simulink model "GHV_open_VarialbeMass_toolbox"  (R2023b)
settings: Solver=VariableStepAuto  StartTime=0.0  StopTime=10  FixedStep=0.0000001  MaxStep=0.001  RelTol=1e-3
InitFcn:
  | run('init.m')
values from neighbouring files (symbols this model uses):
  engine_enable = 1    [GHV_Configuration.m]
  GHV_cfg = struct()    [GHV_Configuration.m]
libraries: simulink_extras x3, aerolibtransform2 x3, aerolibasang x3, shared6dof x1, aerolibatmos2 x1
settings Model: SimulationMode=accelerator  Creator=Admin  LastModifiedBy=Admin
settings SolverCC: AllowMultiTaskInputOutput=on  ZeroCrossControl=EnableAll  ZeroCrossAlgorithm=Adaptive  AutoInsertRateTranBlk=on

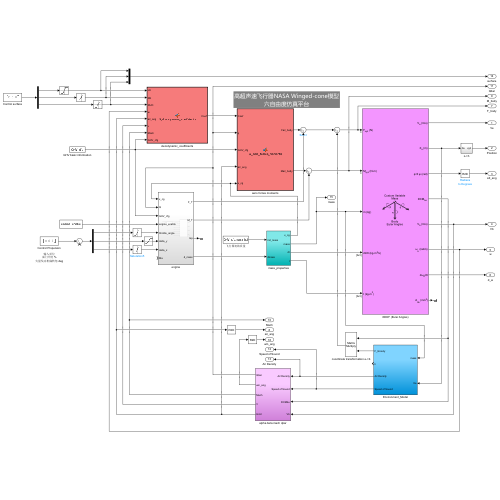
[thumbnail: Simulink's stored preview of the top-level diagram]
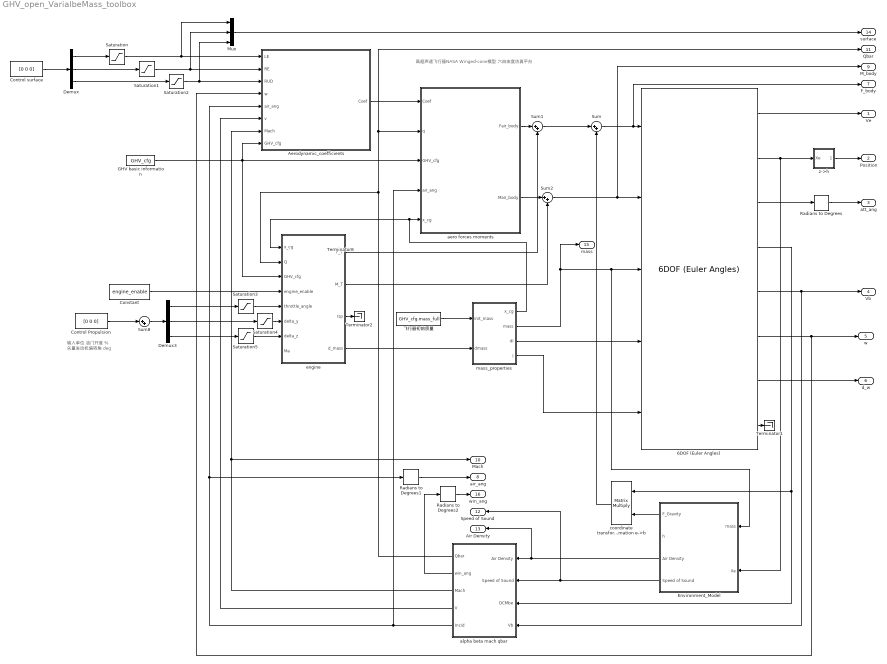
== system GHV_open_VarialbeMass_toolbox ==
  note: 高超声速飞行器NASA Winged-cone模型
      | 六自由度仿真平台
  note: 输入单位
      | 油门开度 %
      | 矢量发动机偏转角 deg
  6DOF (Euler Angles) : shared6dof/6DOF (Euler Angles)  units=Metric (MKS)  mtype=Custom Variable  rep=Euler Angles  xme_0=Position_init  Vm_0=Speed_init  eul_0=Euler_init  pm_0=Omega_init  mass_0=GHV_cfg.mass_full  mass_e=0.5  mass_f=2.0  inertia=GHV_cfg.J  inertia_e=eye(3)  inertia_f=2*eye(3)  k_quat=1.0  vre_flag=off  abi_flag=off  aMode=0  xme_statename=''  Vm_statename=''  eul_statename=''  quat_statename=''  pm_statename=''  mass_statename=''
  Aerodynamic_coefficients : MATLAB Function  TreatAsAtomicUnit=on
  Constant : Constant  Value=engine_enable
  Control Propulsion : Constant  Value=[0 0 0]
  Control surface : Constant  Value=[0 0 0]
  Demux : Demux  Outputs=3
  Demux3 : Demux  Outputs=3
  Environment_Model : Subsystem
  GHV basic information : Constant  Value=GHV_cfg  VectorParams1D=off  OutDataTypeStr=Bus: slBus1
  Mux : Mux  Inputs=3
  Radians to Degrees : simulink_extras/Transformations/Radians to Degrees
  Radians to Degrees1 : simulink_extras/Transformations/Radians to Degrees
  Radians to Degrees2 : simulink_extras/Transformations/Radians to Degrees
  Saturation : Saturate  UpperLimit=30  LowerLimit=-30
  Saturation1 : Saturate  UpperLimit=30  LowerLimit=-30
  Saturation2 : Saturate  UpperLimit=30  LowerLimit=-30
  Saturation3 : Saturate  UpperLimit=52.5  LowerLimit=0  ZeroCross=off
  Saturation4 : Saturate  UpperLimit=10  LowerLimit=-10  ZeroCross=off
  Saturation5 : Saturate  UpperLimit=10  LowerLimit=-10  ZeroCross=off
  Sum{,1..2,8} (4 alike) : Sum  Inputs=|++
  Terminator1 : Terminator
  Terminator2 : Terminator
  Terminator8 : Terminator
  aero forces moments : MATLAB Function  TreatAsAtomicUnit=on
  alpha beta mach qbar : Subsystem
  coordinate transformation e->b : Product  Multiplication=Matrix(*)
  engine : Subsystem
  mass_properties : Subsystem
  z->h : Subsystem
  飞行器初始质量 : Constant  Value=GHV_cfg.mass_full
  Ve : Outport
  Position : Outport  Port=2
  att_ang : Outport  Port=3
  Vb : Outport  Port=4
  w : Outport  Port=5
  d_w : Outport  Port=6
  F_body : Outport  Port=7
  air_ang : Outport  Port=8
  M_body : Outport  Port=9
  Mach : Outport  Port=10
  Qbar : Outport  Port=11
  Speed of Sound : Outport  Port=12
  Air Density : Outport  Port=13
  surface : Outport  Port=14
  mass : Outport  Port=15
  win_ang : Outport  Port=16
  wires:
  aero forces moments/1(Fair_body) -> Sum1/1
  aero forces moments/2(Mair_body) -> Sum2/1
  Environment_Model/1(F_Gravity) -> coordinate transformation e->b/2
  6DOF (Euler Angles)/4 -> coordinate transformation e->b/1, alpha beta mach qbar/3(DCMbe)
  Sum/1 -> F_body/1, 6DOF (Euler Angles)/1
  coordinate transformation e->b/1 -> Sum/2
  6DOF (Euler Angles)/2 -> z->h/1(Xe), Environment_Model/2(Xe)
  Environment_Model/4(Speed of Sound) -> Speed of Sound/1, alpha beta mach qbar/2(Speed of Sound)
  Environment_Model/3(Air Density) -> Air Density/1, alpha beta mach qbar/1(Air Density)
  6DOF (Euler Angles)/5 -> alpha beta mach qbar/4(Vb), Vb/1
  alpha beta mach qbar/1(Qbar) -> aero forces moments/2(q), Qbar/1, engine/2(Q)
  alpha beta mach qbar/5(Incid) -> Aerodynamic_coefficients/5(air_ang), Radians to Degrees1/1, aero forces moments/4(air_ang)
  alpha beta mach qbar/4(V) -> Aerodynamic_coefficients/6(v)
  alpha beta mach qbar/3(Mach) -> Aerodynamic_coefficients/7(Mach), Mach/1
  6DOF (Euler Angles)/1 -> Ve/1
  6DOF (Euler Angles)/3 -> Radians to Degrees/1
  6DOF (Euler Angles)/7 -> d_w/1
  6DOF (Euler Angles)/8 -> Terminator1/1
  Control surface/1 -> Demux/1
  GHV basic information/1 -> engine/3(GHV_cfg), aero forces moments/3(GHV_cfg), Aerodynamic_coefficients/8(GHV_cfg)
  z->h/1(xyh) -> Position/1
  Radians to Degrees/1 -> att_ang/1
  Radians to Degrees1/1 -> air_ang/1
  Demux/1 -> Saturation/1
  Demux/2 -> Saturation1/1
  Demux/3 -> Saturation2/1
  6DOF (Euler Angles)/6 -> w/1, Aerodynamic_coefficients/4(w)
  Saturation/1 -> Aerodynamic_coefficients/1(LE), Mux/1
  Saturation1/1 -> Aerodynamic_coefficients/2(RE), Mux/2
  Saturation2/1 -> Aerodynamic_coefficients/3(RUD), Mux/3
  飞行器初始质量/1 -> mass_properties/1(init_mass)
  engine/4(d_mass) -> mass_properties/2(dmass)
  mass_properties/2(mass) -> mass/1, 6DOF (Euler Angles)/3, Environment_Model/1(mass)
  mass_properties/3(dI) -> 6DOF (Euler Angles)/4
  mass_properties/4(I) -> 6DOF (Euler Angles)/5
  mass_properties/1(x_cg) -> aero forces moments/5(x_cg), engine/1(x_cg)
  Sum1/1 -> Sum/1
  Sum2/1 -> M_body/1, 6DOF (Euler Angles)/2
  engine/1(F_T) -> Sum1/2
  engine/2(M_T) -> Sum2/2
  engine/3(Isp) -> Terminator2/1
  Mux/1 -> surface/1
  alpha beta mach qbar/2(win_ang) -> Radians to Degrees2/1
  Aerodynamic_coefficients/1(Coef) -> aero forces moments/1(Coef)
  Radians to Degrees2/1 -> win_ang/1
  Saturation5/1 -> engine/7(delta_z)
  Constant/1 -> engine/4(engine_enable)
  Saturation4/1 -> engine/6(delta_y)
  Demux3/2 -> Saturation4/1
  Sum8/1 -> Demux3/1
  Demux3/3 -> Saturation5/1
  Saturation3/1 -> engine/5(throttle_angle)
  Control Propulsion/1 -> Sum8/1
  Demux3/1 -> Saturation3/1

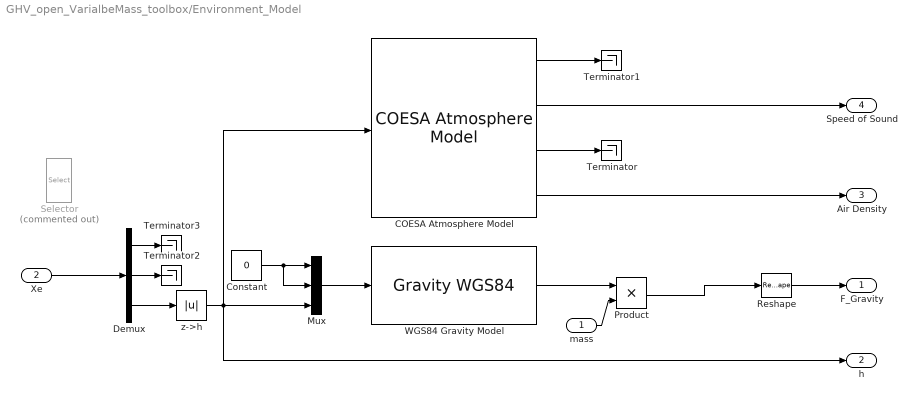
== system GHV_open_VarialbeMass_toolbox/Environment_Model ==
  mass : Inport
  Xe : Inport  Port=2
  COESA Atmosphere Model : aerolibatmos2/COESA Atmosphere Model  units=Metric (MKS)  spec=1976 COESA-extended U.S. Standard Atmosphere  model=Profile  profile_var=High temperature  profile_percent=1%  profile_alt=5 km (16404 ft)  envelope_var=High temperature  envelope_percent=1%  action=Warning
  Constant : Constant  Value=0
  Demux : Demux  Outputs=3
  Mux : Mux  Inputs=3
  Product : Product
  Reshape : Reshape
  Selector : Selector  Commented=on  InputPortWidth=3  IndexOptions=Index vector (dialog)  Indices=[3]  OutputSizes=1
  Terminator{,1..3} (4 alike) : Terminator
  "WGS84 Gravity Model  " : GravityWGS84  action=None
  z->h : Abs  SaturateOnIntegerOverflow=off
  F_Gravity : Outport
  h : Outport  Port=2
  Air Density : Outport  Port=3
  Speed of Sound : Outport  Port=4
  wires:
  Product/1 -> Reshape/1
  Constant/1 -> Mux/2, Mux/1
  z->h/1 -> h/1, COESA Atmosphere Model/1, Mux/3
  Mux/1 -> "WGS84 Gravity Model  "/1
  COESA Atmosphere Model/1 -> Terminator1/1
  COESA Atmosphere Model/2 -> Speed of Sound/1
  COESA Atmosphere Model/3 -> Terminator/1
  "WGS84 Gravity Model  "/1 -> Product/1
  COESA Atmosphere Model/4 -> Air Density/1
  Reshape/1 -> F_Gravity/1
  Xe/1 -> Demux/1
  Demux/3 -> z->h/1
  Demux/2 -> Terminator2/1
  Demux/1 -> Terminator3/1
  mass/1 -> Product/2

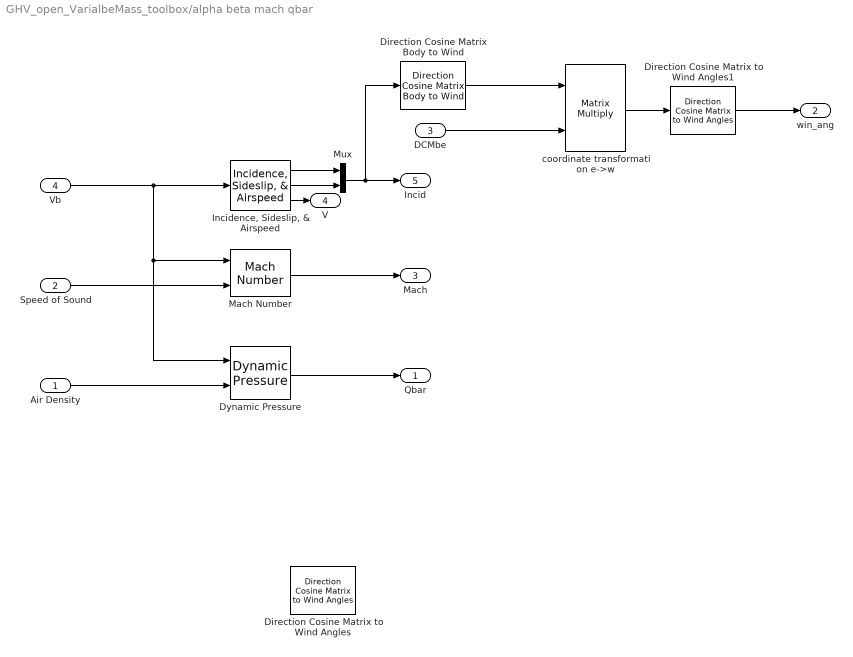
== system GHV_open_VarialbeMass_toolbox/alpha beta mach qbar ==
  Air Density : Inport
  Speed of Sound : Inport  Port=2
  DCMbe : Inport  Port=3
  Vb : Inport  Port=4
  Direction Cosine Matrix Body to Wind : aerolibtransform2/Direction Cosine Matrix Body to Wind
  Direction Cosine Matrix to Wind Angles : aerolibtransform2/Direction Cosine Matrix to Wind Angles  action=None  tolerance=eps(2)
  Direction Cosine Matrix to Wind Angles1 : aerolibtransform2/Direction Cosine Matrix to Wind Angles  action=None  tolerance=eps(2)
  Dynamic Pressure : aerolibasang/Dynamic Pressure
  "Incidence, Sideslip, & Airspeed" : aerolibasang/Incidence, Sideslip, & Airspeed
  Mach Number : aerolibasang/Mach Number
  Mux : Mux  Inputs=2
  coordinate transformation e->w : Product  Multiplication=Matrix(*)
  Qbar : Outport
  win_ang : Outport  Port=2
  Mach : Outport  Port=3
  V : Outport  Port=4
  Incid : Outport  Port=5
  wires:
  Speed of Sound/1 -> Mach Number/2
  Mach Number/1 -> Mach/1
  "Incidence, Sideslip, & Airspeed"/2 -> Mux/2
  Vb/1 -> Dynamic Pressure/1, Mach Number/1, "Incidence, Sideslip, & Airspeed"/1
  Dynamic Pressure/1 -> Qbar/1
  Mux/1 -> Direction Cosine Matrix Body to Wind/1, Incid/1
  "Incidence, Sideslip, & Airspeed"/1 -> Mux/1
  Air Density/1 -> Dynamic Pressure/2
  "Incidence, Sideslip, & Airspeed"/3 -> V/1
  DCMbe/1 -> coordinate transformation e->w/2
  Direction Cosine Matrix Body to Wind/1 -> coordinate transformation e->w/1
  coordinate transformation e->w/1 -> Direction Cosine Matrix to Wind Angles1/1
  Direction Cosine Matrix to Wind Angles1/1 -> win_ang/1

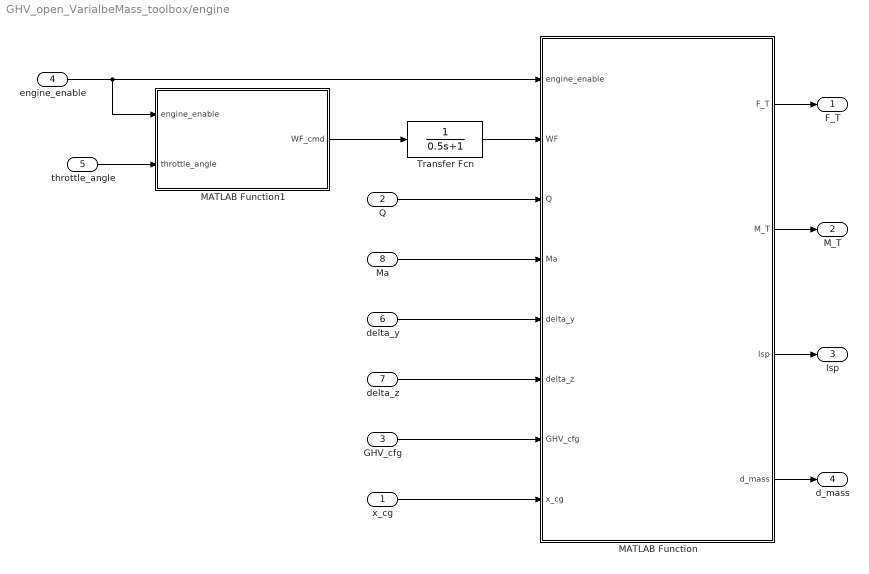
== system GHV_open_VarialbeMass_toolbox/engine ==
  x_cg : Inport
  Q : Inport  Port=2
  GHV_cfg : Inport  Port=3
  engine_enable : Inport  Port=4
  throttle_angle : Inport  Port=5
  delta_y : Inport  Port=6
  delta_z : Inport  Port=7
  Ma : Inport  Port=8
  MATLAB Function : MATLAB Function  TreatAsAtomicUnit=on
  MATLAB Function1 : MATLAB Function  TreatAsAtomicUnit=on
  Transfer Fcn : TransferFcn  Denominator=[0.5 1]
  F_T : Outport
  M_T : Outport  Port=2
  Isp : Outport  Port=3
  d_mass : Outport  Port=4
  wires:
  delta_y/1 -> MATLAB Function/5(delta_y)
  GHV_cfg/1 -> MATLAB Function/7(GHV_cfg)
  Ma/1 -> MATLAB Function/4(Ma)
  delta_z/1 -> MATLAB Function/6(delta_z)
  Transfer Fcn/1 -> MATLAB Function/2(WF)
  MATLAB Function1/1(WF_cmd) -> Transfer Fcn/1
  Q/1 -> MATLAB Function/3(Q)
  MATLAB Function/3(Isp) -> Isp/1
  MATLAB Function/2(M_T) -> M_T/1
  MATLAB Function/1(F_T) -> F_T/1
  x_cg/1 -> MATLAB Function/8(x_cg)
  engine_enable/1 -> MATLAB Function1/1(engine_enable), MATLAB Function/1(engine_enable)
  throttle_angle/1 -> MATLAB Function1/2(throttle_angle)
  MATLAB Function/4(d_mass) -> d_mass/1

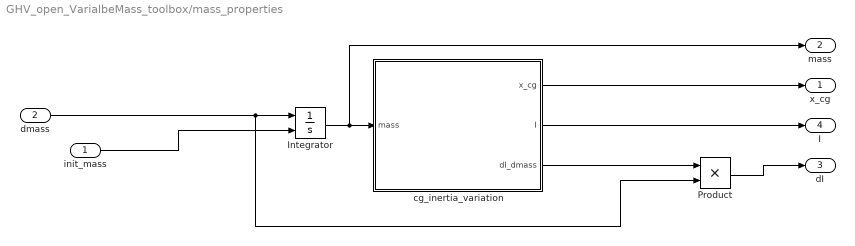
== system GHV_open_VarialbeMass_toolbox/mass_properties ==
  init_mass : Inport
  dmass : Inport  Port=2
  Integrator : Integrator  InitialConditionSource=external
  Product : Product
  cg_inertia_variation : MATLAB Function  TreatAsAtomicUnit=on
  x_cg : Outport
  mass : Outport  Port=2
  dI : Outport  Port=3
  I : Outport  Port=4
  wires:
  Integrator/1 -> mass/1, cg_inertia_variation/1(mass)
  init_mass/1 -> Integrator/2
  cg_inertia_variation/3(dI_dmass) -> Product/1
  dmass/1 -> Product/2, Integrator/1
  cg_inertia_variation/2(I) -> I/1
  cg_inertia_variation/1(x_cg) -> x_cg/1
  Product/1 -> dI/1

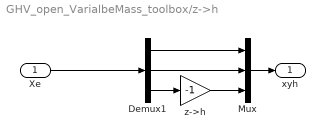
== system GHV_open_VarialbeMass_toolbox/z->h ==
  Xe : Inport
  Demux1 : Demux  Outputs=3
  Mux : Mux  Inputs=3
  z->h : Gain  Gain=-1
  xyh : Outport
  wires:
  z->h/1 -> Mux/3
  Demux1/2 -> Mux/2
  Demux1/3 -> z->h/1
  Demux1/1 -> Mux/1
  Xe/1 -> Demux1/1
  Mux/1 -> xyh/1

== matlab function GHV_open_VarialbeMass_toolbox/Aerodynamic_coefficients ==
  data: LE input; Coef output; RE input; RUD input; w input; air_ang input; v input; Mach input; GHV_cfg input
function Coef = S_Aerodynamic_coefficients(LE, RE, RUD, w, air_ang,v, Mach, GHV_cfg)
    Coef = zeros(6, 1);
    Coef = Aerodynamic_coefficients(LE, RE, RUD, air_ang, v, w, Mach, GHV_cfg);

end

== matlab function GHV_open_VarialbeMass_toolbox/mass_properties/cg_inertia_variation ==
  data: mass input; x_cg output; I output; dI_dmass output
function [x_cg, I, dI_dmass] = S_cg_inertia_variation(mass)

     [x_cg, I, dI_dmass] = cg_inertia_variation(mass);
     
end

== matlab function GHV_open_VarialbeMass_toolbox/aero forces moments ==
  data: Coef input; q input; GHV_cfg input; air_ang input; x_cg input; Fair_body output; Mair_body output
function [Fair_body, Mair_body] = S_aero_forces_moments(Coef, q, GHV_cfg, air_ang, x_cg)

    Fair_body = zeros(3, 1); %#ok<PREALL>
    Mair_body = zeros(3, 1); %#ok<PREALL>
    [Fair_body, Mair_body] = aero_forces_moments(Coef, q, GHV_cfg, x_cg, air_ang);

end

== matlab function GHV_open_VarialbeMass_toolbox/engine/MATLAB Function ==
  data: engine_enable input; F_T output; WF input; Q input; Ma input; delta_y input; delta_z input; GHV_cfg input; x_cg input; M_T output; Isp output; d_mass output
function [F_T, M_T, Isp, d_mass] = S_thrust_vectoring_engine(engine_enable, WF, Q, Ma, delta_y, delta_z, GHV_cfg, x_cg)

    F_T = zeros(3, 1); %#ok<PREALL>
    M_T = zeros(3, 1); %#ok<PREALL>
    [F_T, M_T, Isp, d_mass] = thrust_vectoring_engine(engine_enable, WF, Q, Ma, delta_y, delta_z, GHV_cfg, x_cg);

end

== matlab function GHV_open_VarialbeMass_toolbox/engine/MATLAB Function1 ==
  data: engine_enable input; WF_cmd output; throttle_angle input
function WF_cmd = S_throttle_lever_model(engine_enable, throttle_angle)

    WF_cmd = throttle_lever_model(engine_enable, throttle_angle);

end
